simulink model "model_schwab2"  (R2018b)
settings: Solver=VariableStepAuto  StartTime=0.0  StopTime=10  FixedStep=Ts/10  MaxStep=Ts/10
values from neighbouring files (symbols this model uses):
  A = [0 g/h ; 1 0]    [schwab.m]
  B = [1 ; 0]    [schwab.m]
  bike_params = [g h b a lambda c m]    [schwab.m]
  C = [C1*v C2*v^2]    [schwab.m]
  C1 = a/(b*h)    [schwab.m]    (also in schwab_matlab_block.m = [C111 C112)
  C2 = 1/(b*h)    [schwab.m]
  D = 0    [schwab.m]
  D_steering_position = 0    [schwab.m]
  I_steering_position = 30    [schwab.m]
  initial_roll = deg2rad(0.05)    [schwab.m]
  initial_rollrate = deg2rad(0)    [schwab.m]
  initial_steering = deg2rad(0)    [schwab.m]
  K_feedforward_steering = 0    [schwab.m]
  lqr_gains = zeros(length(velocity_lqr),1+size(A,1))    [lqr_design.m]
  nonlinear_model = 0    [schwab.m]
  num_tf_steering = [253.4]    [schwab.m]
  P_steering_position = 30    [schwab.m]
  Ts = 0.01    [schwab.m]
  uneven_mass = 0    [schwab.m]
  v = 4    [schwab.m]    (also in schwab_matlab_block.m = 0)
  velocity_lqr = [v - 0.1 , v , v + 0.1]    [lqr_design.m]
undefined symbols (not defined in the file or in its folder): A_front, B_front, ba, bb, C_front, D_front
libraries: simulink_extras x8, simulink x2
settings Model: Creator=Boaz Ash  LastModifiedBy=maximef
settings DebuggingCC: UnconnectedInputMsg=none  UnconnectedOutputMsg=none  UnconnectedLineMsg=none  LibraryContextMissingDiagnostic=none
settings SFSimCC: SimUseLocalCustomCode=off
settings RTWCC: RTWUseLocalCustomCode=off

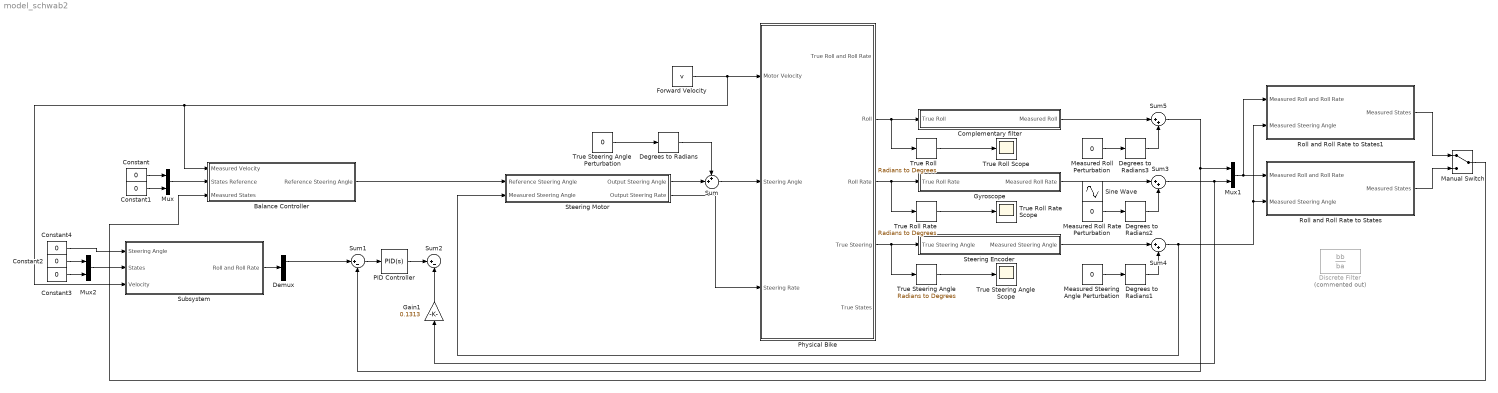
== system model_schwab2 ==
  Balance Controller : Subsystem  SystemSampleTime=Ts
  Complementary filter : Subsystem  TreatAsAtomicUnit=on  SystemSampleTime=Ts
  Constant{,1..4} (5 alike) : Constant  Value=0
  Degrees to Radians{,1..3} (4 alike) : simulink_extras/Transformations/Degrees to Radians
  Demux : Demux  Outputs=2
  Discrete Filter : DiscreteFilter  Commented=on  Numerator=bb  Denominator=ba  SampleTime=Ts
  Forward Velocity : Constant  Value=v
  Gain1 : Gain  Gain=0.1313
  Gyroscope : Subsystem  TreatAsAtomicUnit=on  SystemSampleTime=Ts
  Manual Switch : ManualSwitch
  Measured Roll Perturbation : Constant  Value=0
  Measured Roll Rate Perturbation : Constant  Value=0
  Measured Steering Angle Perturbation : Constant  Value=0
  Mux : Mux  Inputs=2
  Mux1 : Mux  Inputs=2
  Mux2 : Mux  Inputs=2
  PID Controller : simulink/Continuous/PID Controller  Controller=PID  Form=Parallel  TimeDomain=Continuous-time  SampleTime=-1  IntegratorMethod=Forward Euler  FilterMethod=Forward Euler  ControllerParametersSource=internal  P=3.937  I=1.904  D=0  UseFilter=on  N=100  TunerSelectOption=Transfer Function Based (PID Tuner App)  InitialConditionSource=internal  InitialConditionForIntegrator=0  InitialConditionForFilter=0  DifferentiatorICPrevScaledInput=0  ExternalReset=none  TrackingMode=off  Kt=1  LimitOutput=off  UpperSaturationLimit=inf  LowerSaturationLimit=-inf  LinearizeAsGain=on  AntiWindupMode=none  Kb=1  POutMin=[]  POutMax=[]  IOutMin=[]  IOutMax=[]  DOutMin=[]  DOutMax=[]  NOutMin=[]  NOutMax=[]  SumOutMin=[]  SumOutMax=[]  SaturationOutMin=[]  SaturationOutMax=[]  PParamMin=[]  PParamMax=[]  IParamMin=[]  IParamMax=[]  DParamMin=[]  DParamMax=[]  NParamMin=[]  NParamMax=[]  KbParamMin=[]  KbParamMax=[]  KtParamMin=[]  KtParamMax=[]  KbOutMin=[]  KbOutMax=[]  KtOutMin=[]  KtOutMax=[]  IntegratorOutMin=[]  IntegratorOutMax=[]  FilterOutMin=[]  FilterOutMax=[]  SumI1OutMin=[]  SumI1OutMax=[]  SumI2OutMin=[]  SumI2OutMax=[]  SumI3OutMin=[]  SumI3OutMax=[]  SumI4OutMin=[]  SumI4OutMax=[]  SumDOutMin=[]  SumDOutMax=[]  DifferentiatorOutMin=[]  DifferentiatorOutMax=[]  FilterDiffOutCoefMin=[]  FilterDiffOutCoefMax=[]  ReciprocalOutMin=[]  ReciprocalOutMax=[]  SumDenOutMin=[]  SumDenOutMax=[]  SumNumOutMin=[]  SumNumOutMax=[]  DivideOutMin=[]  DivideOutMax=[]  IntegratorContinuousStateAttributes=''  IntegratorStateMustResolveToSignalObject=off  IntegratorRTWStateStorageClass=Auto  FilterContinuousStateAttributes=''  FilterStateMustResolveToSignalObject=off  FilterRTWStateStorageClass=Auto  ParallelPVariant=InternalParameters  IdealPVariant=Disabled  IVariant=InternalParameters  DVariant=InternalParameters  IntegratorVariant=Continuous  SatVariant=Disabled  AWVariant=Passthrough  PCopyVariant=Disabled  TRVariant=Disabled  FdbkBlocksVariant=Forward  IdealPFdbkVariant=Disabled  SatFdbkVariant=Disabled  DerivativeFilterVariant=ContFilter  NVariant=InternalParameters  NCopyVariant=Disabled  FilterICVariant=InternalICsFilter  IntegratorICVariant=InternalICs  ExternalResetVariant=Disabled  TRSumVariant=Passthrough  SumFdbkVariant=Disabled  SumVariant=Sum_PID
  Physical Bike : Subsystem
  Roll and Roll Rate to States : Subsystem
  Roll and Roll Rate to States1 : Subsystem
  Sine Wave : Sin  Amplitude=0.5  Frequency=2*pi*1  SampleTime=0
  Steering Encoder : Subsystem  TreatAsAtomicUnit=on  SystemSampleTime=Ts
  Steering Motor : Subsystem
  Subsystem : Subsystem
  Sum : Sum  Inputs=++|
  Sum1 : Sum  Inputs=|+-
  Sum2 : Sum  Inputs=|+-
  Sum3 : Sum  Inputs=|++
  Sum4 : Sum  Inputs=|++
  Sum5 : Sum  Inputs=|++
  True Roll : simulink_extras/Transformations/Radians to Degrees
  True Roll Rate : simulink_extras/Transformations/Radians to Degrees
  True Roll Rate Scope : Scope
  True Roll Scope : Scope
  True Steering Angle : simulink_extras/Transformations/Radians to Degrees
  True Steering Angle Perturbation : Constant  Value=0
  True Steering Angle Scope : Scope
  wires:
  Sum1/1 -> PID Controller/1
  PID Controller/1 -> Sum2/1
  Sum/1 -> Physical Bike/2(Steering Angle)
  Constant/1 -> Mux/1
  True Steering Angle Perturbation/1 -> Degrees to Radians/1
  Mux1/1 -> Roll and Roll Rate to States1/1(Measured Roll and Roll Rate), Roll and Roll Rate to States/1(Measured Roll and Roll Rate)
  Manual Switch/1 -> Balance Controller/3(Measured States)
  Mux/1 -> Balance Controller/2(States Reference)
  Balance Controller/1(Reference Steering Angle) -> Steering Motor/1(Reference Steering Angle)
  Demux/1 -> Sum1/1
  Gain1/1 -> Sum2/2
  Sum5/1 -> Sum1/2, Mux1/1
  Constant1/1 -> Mux/2
  Measured Steering Angle Perturbation/1 -> Degrees to Radians1/1
  True Steering Angle/1 -> True Steering Angle Scope/1
  Physical Bike/4(True Steering) -> Steering Encoder/1(True Steering Angle), True Steering Angle/1
  Steering Encoder/1(Measured Steering Angle) -> Sum4/1
  Degrees to Radians1/1 -> Sum4/2
  Measured Roll Rate Perturbation/1 -> Degrees to Radians2/1
  True Roll Rate/1 -> True Roll Rate Scope/1
  Degrees to Radians2/1 -> Sum3/2
  Physical Bike/3(Roll Rate) -> Gyroscope/1(True Roll Rate), True Roll Rate/1
  Measured Roll Perturbation/1 -> Degrees to Radians3/1
  Complementary filter/1(Measured Roll) -> Sum5/1
  True Roll/1 -> True Roll Scope/1
  Degrees to Radians3/1 -> Sum5/2
  Physical Bike/2(Roll) -> Complementary filter/1(True Roll), True Roll/1
  Sum3/1 -> Mux1/2, Gain1/1
  Sum4/1 -> Steering Motor/2(Measured Steering Angle), Roll and Roll Rate to States1/2(Measured Steering Angle), Roll and Roll Rate to States/2(Measured Steering Angle)
  Gyroscope/1(Measured Roll Rate) -> Sum3/1
  Subsystem/1(Roll and Roll Rate) -> Demux/1
  Constant3/1 -> Mux2/2
  Mux2/1 -> Subsystem/2(States)
  Constant2/1 -> Mux2/1
  Constant4/1 -> Subsystem/1(Steering Angle)
  Roll and Roll Rate to States1/1(Measured States) -> Manual Switch/1
  Roll and Roll Rate to States/1(Measured States) -> Manual Switch/2
  Steering Motor/1(Output Steering Angle) -> Sum/2
  Degrees to Radians/1 -> Sum/1
  Steering Motor/2(Output Steering Rate) -> Physical Bike/3(Steering Rate)
  Forward Velocity/1 -> Physical Bike/1(Motor Velocity), Subsystem/3(Velocity), Balance Controller/1(Measured Velocity)

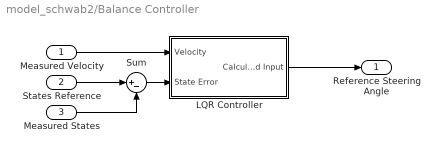
== system model_schwab2/Balance Controller ==
  Measured Velocity : Inport
  States Reference : Inport  Port=2
  Measured States : Inport  Port=3
  LQR Controller : Subsystem  TreatAsAtomicUnit=on  SystemSampleTime=Ts
  Sum : Sum  Inputs=|+-
  Reference Steering Angle : Outport
  wires:
  Sum/1 -> LQR Controller/2(State Error)
  Measured States/1 -> Sum/2
  LQR Controller/1(Calculated Input) -> Reference Steering Angle/1
  Measured Velocity/1 -> LQR Controller/1(Velocity)
  States Reference/1 -> Sum/1

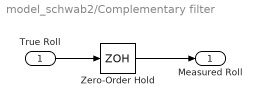
== system model_schwab2/Complementary filter ==
  True Roll : Inport
  Zero-Order Hold : ZeroOrderHold  SampleTime=Ts
  Measured Roll : Outport
  wires:
  True Roll/1 -> Zero-Order Hold/1
  Zero-Order Hold/1 -> Measured Roll/1

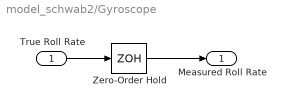
== system model_schwab2/Gyroscope ==
  True Roll Rate : Inport
  Zero-Order Hold : ZeroOrderHold  SampleTime=Ts
  Measured Roll Rate : Outport
  wires:
  True Roll Rate/1 -> Zero-Order Hold/1
  Zero-Order Hold/1 -> Measured Roll Rate/1

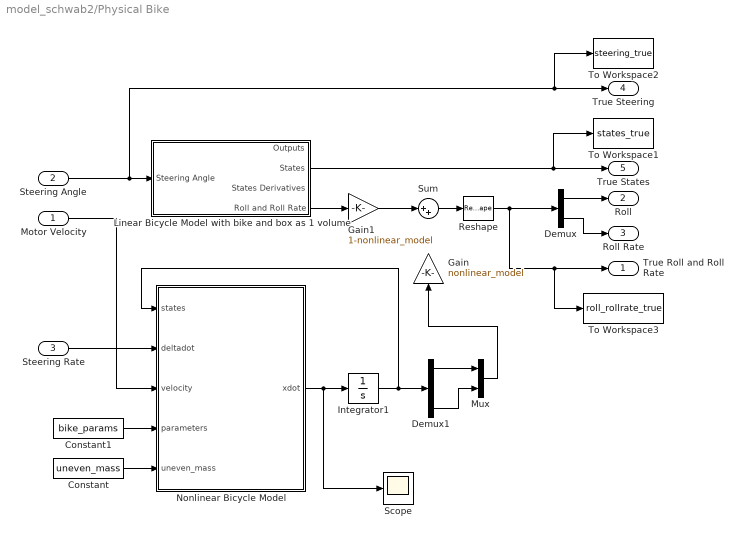
== system model_schwab2/Physical Bike ==
  Motor Velocity : Inport
  Steering Angle : Inport  Port=2
  Steering Rate : Inport  Port=3
  Constant : Constant  Value=uneven_mass
  Constant1 : Constant  Value=bike_params
  Demux : Demux  Outputs=2
  Demux1 : Demux  Outputs=3
  Gain : Gain  Gain=nonlinear_model
  Gain1 : Gain  Gain=1-nonlinear_model
  Integrator1 : Integrator  InitialCondition=[initial_roll initial_rollrate initial_steering]
  Linear Bicycle Model with bike and box as 1 volume : Subsystem
  Mux : Mux  Inputs=2
  Nonlinear Bicycle Model : MATLAB Function  TreatAsAtomicUnit=on
  Reshape : Reshape
  Scope : Scope
  Sum : Sum  Inputs=|++
  To Workspace1 : ToWorkspace  VariableName=states_true  SaveFormat=Timeseries  SampleTime=-1
  To Workspace2 : ToWorkspace  VariableName=steering_true  SaveFormat=Timeseries  SampleTime=-1
  To Workspace3 : ToWorkspace  VariableName=roll_rollrate_true  SaveFormat=Timeseries  SampleTime=-1
  True Roll and Roll Rate : Outport
  Roll : Outport  Port=2
  Roll Rate : Outport  Port=3
  True Steering : Outport  Port=4
  True States : Outport  Port=5
  wires:
  Steering Angle/1 -> Linear Bicycle Model with bike and box as 1 volume/1(Steering Angle), To Workspace2/1, True Steering/1
  Motor Velocity/1 -> Nonlinear Bicycle Model/3(velocity)
  Linear Bicycle Model with bike and box as 1 volume/2(States) -> True States/1, To Workspace1/1
  Demux/1 -> Roll/1
  Linear Bicycle Model with bike and box as 1 volume/4(Roll and Roll Rate) -> Gain1/1
  Reshape/1 -> To Workspace3/1, True Roll and Roll Rate/1, Demux/1
  Demux/2 -> Roll Rate/1
  Nonlinear Bicycle Model/1(xdot) -> Integrator1/1, Scope/1
  Integrator1/1 -> Demux1/1, Nonlinear Bicycle Model/1(states)
  Constant/1 -> Nonlinear Bicycle Model/5(uneven_mass)
  Constant1/1 -> Nonlinear Bicycle Model/4(parameters)
  Steering Rate/1 -> Nonlinear Bicycle Model/2(deltadot)
  Demux1/1 -> Mux/1
  Demux1/3 -> Mux/2
  Sum/1 -> Reshape/1
  Gain1/1 -> Sum/1
  Mux/1 -> Gain/1

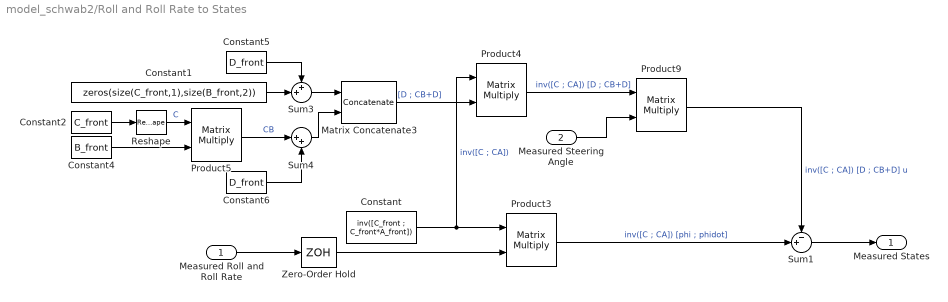
== system model_schwab2/Roll and Roll Rate to States ==
  Measured Roll and Roll Rate : Inport
  Measured Steering Angle : Inport  Port=2
  Constant : Constant  Value=inv([C_front ; C_front*A_front])
  Constant1 : Constant  Value=zeros(size(C_front,1),size(B_front,2))
  Constant2 : Constant  Value=C_front
  Constant4 : Constant  Value=B_front
  Constant5 : Constant  Value=D_front
  Constant6 : Constant  Value=D_front
  Matrix Concatenate3 : Concatenate  Mode=Multidimensional array
  Product{3..5,9} (4 alike) : Product  SCDEnableBlockLinearizationSpecification=on  Multiplication=Matrix(*)
  Reshape : Reshape  OutputDimensionality=Customize  OutputDimensions=[size(C,1),size(C,2)]
  Sum1 : Sum  Inputs=-+|
  Sum3 : Sum  Inputs=++|
  Sum4 : Sum  Inputs=|++
  Zero-Order Hold : ZeroOrderHold  SampleTime=Ts
  Measured States : Outport
  wires:
  Constant2/1 -> Reshape/1
  Constant/1 -> Product4/1, Product3/1  "inv([C ; CA])"
  Measured Roll and Roll Rate/1 -> Zero-Order Hold/1
  Product3/1 -> Sum1/2  "inv([C ; CA]) [phi ; phidot]"
  Matrix Concatenate3/1 -> Product4/2  "[D ; CB+D]"
  Product5/1 -> Sum4/1  "CB"
  Constant4/1 -> Product5/2
  Constant1/1 -> Sum3/2
  Product4/1 -> Product9/1  "inv([C ; CA]) [D ; CB+D]"
  Measured Steering Angle/1 -> Product9/2
  Product9/1 -> Sum1/1  "inv([C ; CA]) [D ; CB+D] u"
  Sum1/1 -> Measured States/1
  Zero-Order Hold/1 -> Product3/2
  Constant6/1 -> Sum4/2
  Constant5/1 -> Sum3/1
  Sum4/1 -> Matrix Concatenate3/2
  Sum3/1 -> Matrix Concatenate3/1
  Reshape/1 -> Product5/1  "C"

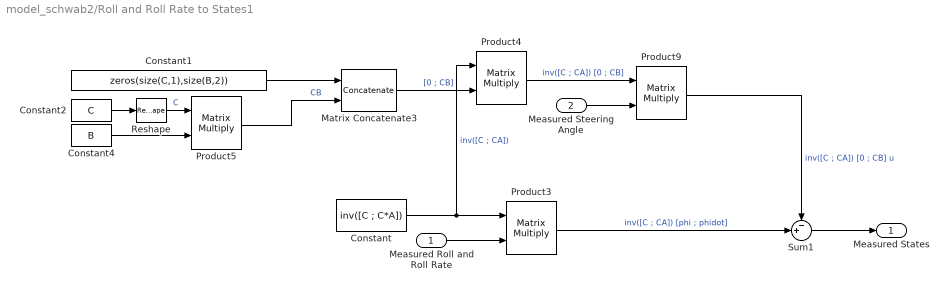
== system model_schwab2/Roll and Roll Rate to States1 ==
  Measured Roll and Roll Rate : Inport
  Measured Steering Angle : Inport  Port=2
  Constant : Constant  Value=inv([C ; C*A])
  Constant1 : Constant  Value=zeros(size(C,1),size(B,2))
  Constant2 : Constant  Value=C
  Constant4 : Constant  Value=B
  Matrix Concatenate3 : Concatenate  Mode=Multidimensional array
  Product{3..5,9} (4 alike) : Product  SCDEnableBlockLinearizationSpecification=on  Multiplication=Matrix(*)
  Reshape : Reshape  OutputDimensionality=Customize  OutputDimensions=[size(C,1),size(C,2)]
  Sum1 : Sum  Inputs=-+|
  Measured States : Outport
  wires:
  Constant2/1 -> Reshape/1
  Constant/1 -> Product4/1, Product3/1  "inv([C ; CA])"
  Product3/1 -> Sum1/2  "inv([C ; CA]) [phi ; phidot]"
  Matrix Concatenate3/1 -> Product4/2  "[0 ; CB]"
  Product5/1 -> Matrix Concatenate3/2  "CB"
  Constant4/1 -> Product5/2
  Product4/1 -> Product9/1  "inv([C ; CA]) [0 ; CB]"
  Measured Steering Angle/1 -> Product9/2
  Product9/1 -> Sum1/1  "inv([C ; CA]) [0 ; CB] u"
  Sum1/1 -> Measured States/1
  Measured Roll and Roll Rate/1 -> Product3/2
  Constant1/1 -> Matrix Concatenate3/1
  Reshape/1 -> Product5/1  "C"

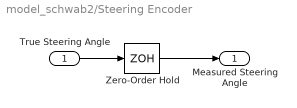
== system model_schwab2/Steering Encoder ==
  True Steering Angle : Inport
  Zero-Order Hold : ZeroOrderHold  SampleTime=Ts
  Measured Steering Angle : Outport
  wires:
  True Steering Angle/1 -> Zero-Order Hold/1
  Zero-Order Hold/1 -> Measured Steering Angle/1

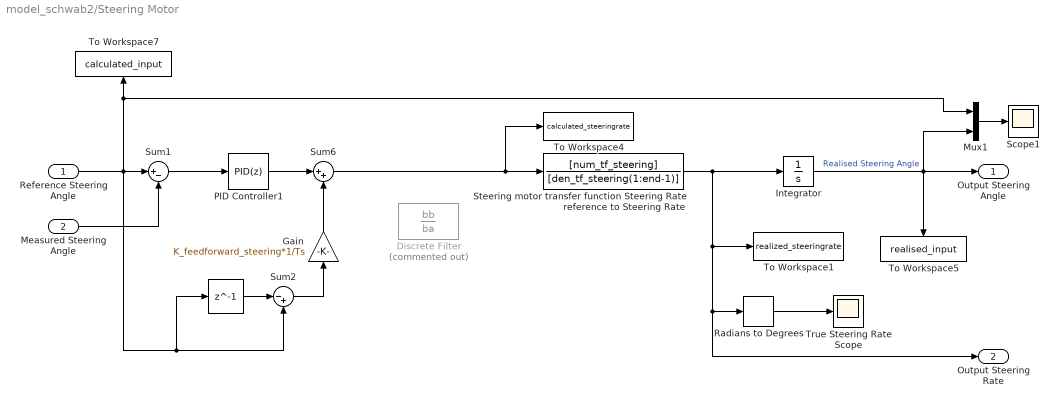
== system model_schwab2/Steering Motor ==
  Reference Steering Angle : Inport
  Measured Steering Angle : Inport  Port=2
  " " : Delay  DelayLength=1  SampleTime=Ts
  Discrete Filter : DiscreteFilter  Commented=on  Numerator=bb  Denominator=ba
  Gain : Gain  Gain=K_feedforward_steering*1/Ts
  Integrator : Integrator  InitialCondition=initial_steering
  Mux1 : Mux  Inputs=2
  PID Controller1 : simulink/Continuous/PID Controller  Controller=PID  Form=Parallel  TimeDomain=Discrete-time  SampleTime=Ts  IntegratorMethod=Forward Euler  FilterMethod=Forward Euler  ControllerParametersSource=internal  P=P_steering_position  I=I_steering_position  D=D_steering_position  UseFilter=off  N=1  TunerSelectOption=Transfer Function Based (PID Tuner App)  InitialConditionSource=internal  InitialConditionForIntegrator=0  InitialConditionForFilter=0  DifferentiatorICPrevScaledInput=0  ExternalReset=none  TrackingMode=off  Kt=1  LimitOutput=off  UpperSaturationLimit=inf  LowerSaturationLimit=-inf  LinearizeAsGain=on  AntiWindupMode=none  Kb=1  POutMin=[]  POutMax=[]  IOutMin=[]  IOutMax=[]  DOutMin=[]  DOutMax=[]  NOutMin=[]  NOutMax=[]  SumOutMin=[]  SumOutMax=[]  SaturationOutMin=[]  SaturationOutMax=[]  PParamMin=[]  PParamMax=[]  IParamMin=[]  IParamMax=[]  DParamMin=[]  DParamMax=[]  NParamMin=[]  NParamMax=[]  KbParamMin=[]  KbParamMax=[]  KtParamMin=[]  KtParamMax=[]  KbOutMin=[]  KbOutMax=[]  KtOutMin=[]  KtOutMax=[]  IntegratorOutMin=[]  IntegratorOutMax=[]  FilterOutMin=[]  FilterOutMax=[]  SumI1OutMin=[]  SumI1OutMax=[]  SumI2OutMin=[]  SumI2OutMax=[]  SumI3OutMin=[]  SumI3OutMax=[]  SumI4OutMin=[]  SumI4OutMax=[]  SumDOutMin=[]  SumDOutMax=[]  DifferentiatorOutMin=[]  DifferentiatorOutMax=[]  FilterDiffOutCoefMin=[]  FilterDiffOutCoefMax=[]  ReciprocalOutMin=[]  ReciprocalOutMax=[]  SumDenOutMin=[]  SumDenOutMax=[]  SumNumOutMin=[]  SumNumOutMax=[]  DivideOutMin=[]  DivideOutMax=[]  IntegratorContinuousStateAttributes=''  IntegratorStateMustResolveToSignalObject=off  IntegratorRTWStateStorageClass=Auto  FilterContinuousStateAttributes=''  FilterStateMustResolveToSignalObject=off  FilterRTWStateStorageClass=Auto  ParallelPVariant=InternalParameters  IdealPVariant=Disabled  IVariant=InternalParameters  DVariant=InternalParameters  IntegratorVariant=Discrete  SatVariant=Disabled  AWVariant=Passthrough  PCopyVariant=Disabled  TRVariant=Disabled  FdbkBlocksVariant=Forward  IdealPFdbkVariant=Disabled  SatFdbkVariant=Disabled  DerivativeFilterVariant=Differentiator  NVariant=Passthrough  NCopyVariant=Disabled_SignalSpec  FilterICVariant=InternalICsDifferentiator  IntegratorICVariant=InternalICs  ExternalResetVariant=Disabled  TRSumVariant=Passthrough  SumFdbkVariant=Disabled  SumVariant=Sum_PID
  Radians to Degrees : simulink_extras/Transformations/Radians to Degrees
  Scope1 : Scope
  Steering motor transfer function Steering Rate reference to Steering Rate : TransferFcn  Numerator=[num_tf_steering]  Denominator=[den_tf_steering(1:end-1)]
  Sum1 : Sum  Inputs=|+-
  Sum2 : Sum  Inputs=|-+
  Sum6 : Sum  Inputs=|++
  To Workspace1 : ToWorkspace  VariableName=realized_steeringrate  SaveFormat=Timeseries  SampleTime=-1
  To Workspace4 : ToWorkspace  VariableName=calculated_steeringrate  SaveFormat=Timeseries  SampleTime=-1
  To Workspace5 : ToWorkspace  VariableName=realised_input  SaveFormat=Timeseries  SampleTime=-1
  To Workspace7 : ToWorkspace  VariableName=calculated_input  SaveFormat=Timeseries  SampleTime=Ts
  True Steering Rate Scope : Scope
  Output Steering Angle : Outport
  Output Steering Rate : Outport  Port=2
  wires:
  Mux1/1 -> Scope1/1
  Reference Steering Angle/1 -> Mux1/1, To Workspace7/1, Sum1/1, Sum2/2, " "/1
  Measured Steering Angle/1 -> Sum1/2
  " "/1 -> Sum2/1
  Sum2/1 -> Gain/1
  Sum1/1 -> PID Controller1/1
  Integrator/1 -> Output Steering Angle/1, Mux1/2, To Workspace5/1  "Realised Steering Angle"
  PID Controller1/1 -> Sum6/1
  Gain/1 -> Sum6/2
  Steering motor transfer function Steering Rate reference to Steering Rate/1 -> Integrator/1, Output Steering Rate/1, Radians to Degrees/1, To Workspace1/1
  Sum6/1 -> Steering motor transfer function Steering Rate reference to Steering Rate/1, To Workspace4/1
  Radians to Degrees/1 -> True Steering Rate Scope/1

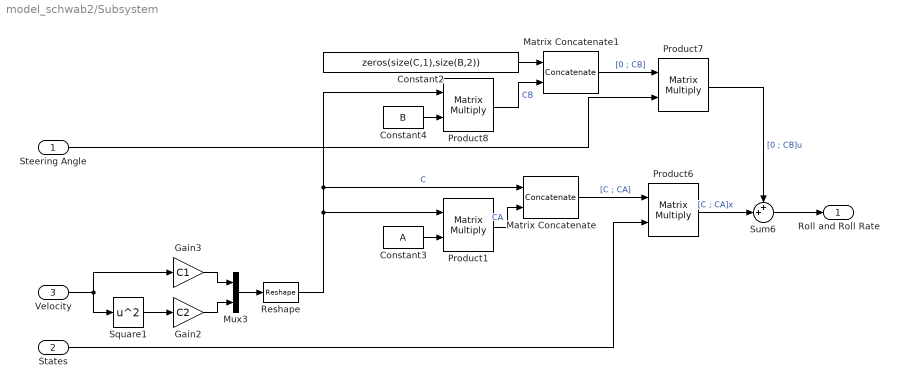
== system model_schwab2/Subsystem ==
  Steering Angle : Inport
  States : Inport  Port=2
  Velocity : Inport  Port=3
  Constant2 : Constant  Value=zeros(size(C,1),size(B,2))
  Constant3 : Constant  Value=A
  Constant4 : Constant  Value=B
  Gain2 : Gain  Gain=C2
  Gain3 : Gain  Gain=C1
  Matrix Concatenate : Concatenate  Mode=Multidimensional array
  Matrix Concatenate1 : Concatenate  Mode=Multidimensional array
  Mux3 : Mux  Inputs=2
  Product{1,6..8} (4 alike) : Product  SCDEnableBlockLinearizationSpecification=on  Multiplication=Matrix(*)
  Reshape : Reshape  OutputDimensionality=Row vector (2-D)
  Square1 : Math  Operator=square  SaturateOnIntegerOverflow=on
  Sum6 : Sum  Inputs=++|
  Roll and Roll Rate : Outport
  wires:
  Product8/1 -> Matrix Concatenate1/2  "CB"
  Product7/1 -> Sum6/1  "[0 ; CB]u"
  Mux3/1 -> Reshape/1
  Constant4/1 -> Product8/2
  Matrix Concatenate1/1 -> Product7/1  "[0 ; CB]"
  Product6/1 -> Sum6/2  "[C ; CA]x"
  Constant3/1 -> Product1/2
  Sum6/1 -> Roll and Roll Rate/1
  Reshape/1 -> Product8/1, Matrix Concatenate/1, Product1/1  "C"
  Matrix Concatenate/1 -> Product6/1  "[C ; CA]"
  Product1/1 -> Matrix Concatenate/2  "CA"
  Gain2/1 -> Mux3/2
  States/1 -> Product6/2
  Gain3/1 -> Mux3/1
  Velocity/1 -> Gain3/1, Square1/1
  Square1/1 -> Gain2/1
  Constant2/1 -> Matrix Concatenate1/1
  Steering Angle/1 -> Product7/2

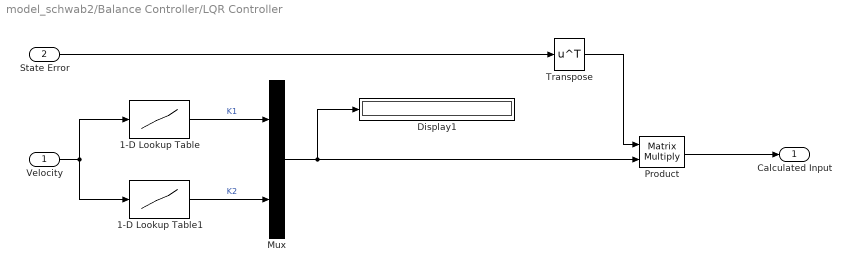
== system model_schwab2/Balance Controller/LQR Controller ==
  Velocity : Inport
  State Error : Inport  Port=2
  1-D Lookup Table : Lookup_n-D  NumberOfTableDimensions=1  BreakpointsForDimension1=velocity_lqr  BreakpointsForDimension2=velocity_lqr  BreakpointsForDimension3=velocity_lqr  BreakpointsForDimension4=velocity_lqr  Table=lqr_gains(:,2)  InternalRulePriority=Speed  RndMeth=Simplest  InputSameDT=on
  1-D Lookup Table1 : Lookup_n-D  NumberOfTableDimensions=1  BreakpointsForDimension1=velocity_lqr  BreakpointsForDimension2=velocity_lqr  BreakpointsForDimension3=velocity_lqr  BreakpointsForDimension4=velocity_lqr  Table=lqr_gains(:,3)  InternalRulePriority=Speed  RndMeth=Simplest  InputSameDT=on
  Display1 : Display
  Mux : Mux  Inputs=2
  Product : Product  Multiplication=Matrix(*)
  Transpose : Math  Operator=transpose  SaturateOnIntegerOverflow=on
  Calculated Input : Outport
  wires:
  1-D Lookup Table/1 -> Mux/1  "K1"
  1-D Lookup Table1/1 -> Mux/2  "K2"
  Velocity/1 -> 1-D Lookup Table1/1, 1-D Lookup Table/1
  Mux/1 -> Product/2, Display1/1
  Transpose/1 -> Product/1
  Product/1 -> Calculated Input/1
  State Error/1 -> Transpose/1

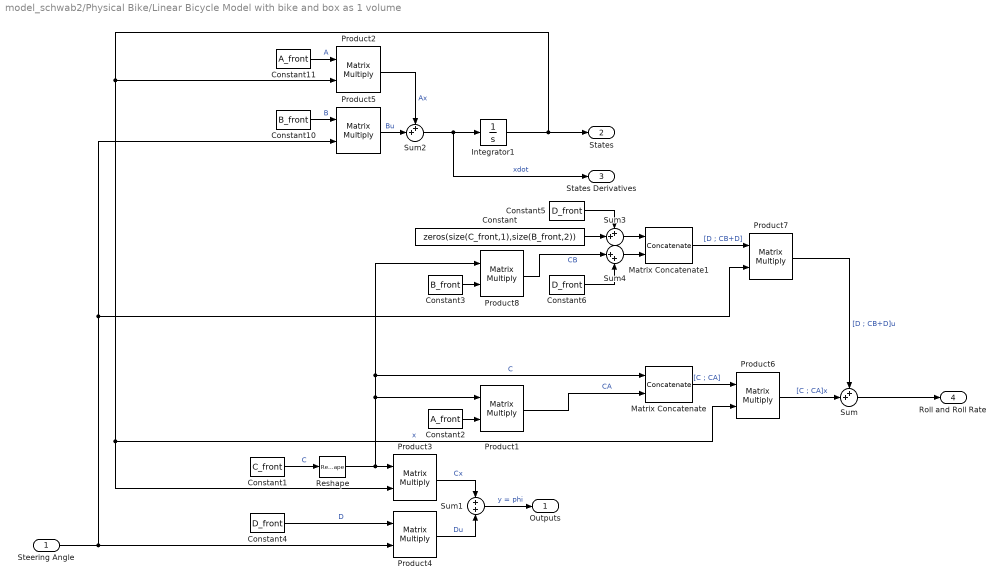
== system model_schwab2/Physical Bike/Linear Bicycle Model with bike and box as 1 volume ==
  Steering Angle : Inport
  Constant : Constant  Value=zeros(size(C_front,1),size(B_front,2))
  Constant1 : Constant  Value=C_front
  Constant10 : Constant  Value=B_front
  Constant11 : Constant  Value=A_front
  Constant2 : Constant  Value=A_front
  Constant3 : Constant  Value=B_front
  Constant4 : Constant  Value=D_front
  Constant5 : Constant  Value=D_front
  Constant6 : Constant  Value=D_front
  Integrator1 : Integrator  InitialCondition=[C_front ; C_front*A_front]\[initial_roll ; initial_rollrate]
  Matrix Concatenate : Concatenate  Mode=Multidimensional array
  Matrix Concatenate1 : Concatenate  Mode=Multidimensional array
  Product{1..8} (8 alike) : Product  SCDEnableBlockLinearizationSpecification=on  Multiplication=Matrix(*)
  Reshape : Reshape  OutputDimensionality=Customize  OutputDimensions=[size(C,1),size(C,2)]
  Sum : Sum  Inputs=++|
  Sum1 : Sum
  Sum2 : Sum  Inputs=++|
  Sum3 : Sum  Inputs=++|
  Sum4 : Sum  Inputs=|++
  Outputs : Outport
  States : Outport  Port=2
  States Derivatives : Outport  Port=3
  Roll and Roll Rate : Outport  Port=4
  wires:
  Reshape/1 -> Product3/1, Product8/1, Matrix Concatenate/1, Product1/1  "C"
  Sum/1 -> Roll and Roll Rate/1
  Constant1/1 -> Reshape/1  "C"
  Matrix Concatenate/1 -> Product6/1  "[C ; CA]"
  Product5/1 -> Sum2/2  "Bu"
  Matrix Concatenate1/1 -> Product7/1  "[D ; CB+D]"
  Constant11/1 -> Product2/1  "A"
  Constant3/1 -> Product8/2
  Product6/1 -> Sum/2  "[C ; CA]x"
  Sum2/1 -> Integrator1/1, States Derivatives/1  "xdot"
  Product2/1 -> Sum2/1  "Ax"
  Product1/1 -> Matrix Concatenate/2  "CA"
  Product8/1 -> Sum4/1  "CB"
  Integrator1/1 -> Product2/2, Product6/2, Product3/2, States/1  "x"
  Sum1/1 -> Outputs/1  "y = phi"
  Constant2/1 -> Product1/2
  Product7/1 -> Sum/1  "[D ; CB+D]u"
  Constant10/1 -> Product5/1  "B"
  Steering Angle/1 -> Product4/2, Product5/2, Product7/2
  Product4/1 -> Sum1/2  "Du"
  Product3/1 -> Sum1/1  "Cx"
  Constant4/1 -> Product4/1  "D"
  Sum3/1 -> Matrix Concatenate1/1
  Constant/1 -> Sum3/2
  Constant5/1 -> Sum3/1
  Sum4/1 -> Matrix Concatenate1/2
  Constant6/1 -> Sum4/2

== matlab function model_schwab2/Physical Bike/Nonlinear Bicycle Model ==
  data: states input; deltadot input; xdot output; velocity input; parameters input; uneven_mass input
function xdot = fcn(states,deltadot,velocity,parameters,uneven_mass)

delta_d=deltadot;
v=velocity;

g=parameters(1);
h=parameters(2);
b=parameters(3);
a=parameters(4);
lambda=parameters(5);
c=parameters(6);
m=parameters(7);

phi=states(1);
delta=states(2);
phi_d=states(3);

J=((m/12)*((c^2)+(b^2)))+(m*(h^2));
% Biaised mass from box mass measurement
% if uneven_mass
%     m = 9.3;
%     d = 0.03;
%     T = m*d*g*cos(phi)/J;
% else
%     T = 0;
% end

% Biaised mass from bike equilibrium measurement
if uneven_mass
    m = 9.3;
    d = 0.07;
    T = m*d*g*cos(phi)/J;
else
    T = 0;
end

xdot1=phi_d;
xdot2=delta_d;
xdot3=(g/h)*tan(phi) - T +((a*v)/(b*h))*sin(lambda)*tan(delta_d)+((h*v^2-g*a*c)/(b*h^2))*sin(lambda)*tan(delta);

xdot=[xdot1 xdot2 xdot3];
